simulink model "PID_simulation_kalman"  (R2015b)
settings: Solver=FixedStepAuto  StartTime=0.0  StopTime=10.0  RelTol=1e-3
values from neighbouring files (symbols this model uses):
  P = (eye(2) - K*C)*Pm    [KF.m]    (also in Kalman_filter_7DOF.m; NEW_PID_4DOF.m = PHI*P*PHI' + EE*K*Rb*K'*EE' + Gd; New_PID.m = PHI*P*PHI' + EE*K*Rb*K'*EE' + Gd; P.mat = [1 0 0 0 0 0 0 0 0 0 0 0 ... (3136 elements, 56x56)])
undefined symbols (not defined in the file or in its folder): sample_time
libraries: dspadpt3 x7
settings Model: Creator=Paul_local  LastModifiedBy=Paul_local

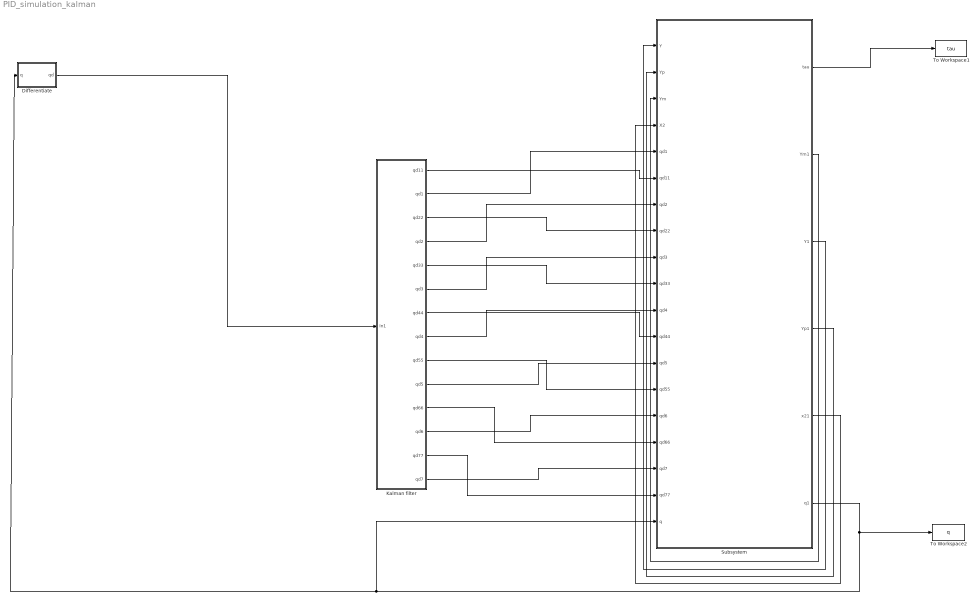
== system PID_simulation_kalman ==
  Differentiate : Subsystem
  Kalman filter : Subsystem
  Subsystem : Subsystem
  To Workspace1 : ToWorkspace  VariableName=tau  SaveFormat=Structure With Time  SampleTime=-1
  To Workspace2 : ToWorkspace  VariableName=q  SaveFormat=Structure With Time  SampleTime=-1
  wires:
  Subsystem/2(Ym1) -> Subsystem/3(Ym)
  Subsystem/5(x21) -> Subsystem/4(X2)
  Subsystem/3(Y1) -> Subsystem/1(Y)
  Subsystem/4(Yp1) -> Subsystem/2(Yp)
  Subsystem/1(tau) -> To Workspace1/1
  Differentiate/1(qd) -> Kalman filter/1(In1)
  Subsystem/6("q1 ") -> To Workspace2/1, Subsystem/19(q), Differentiate/1(q)
  Kalman filter/1(qd11) -> Subsystem/6(qd11)
  Kalman filter/2(qd1) -> Subsystem/5(qd1)
  Kalman filter/3(qd22) -> Subsystem/8(qd22)
  Kalman filter/4(qd2) -> Subsystem/7(qd2)
  Kalman filter/5(qd33) -> Subsystem/10(qd33)
  Kalman filter/6(qd3) -> Subsystem/9(qd3)
  Kalman filter/7(qd44) -> Subsystem/12(qd44)
  Kalman filter/8(qd4) -> Subsystem/11(qd4)
  Kalman filter/9(qd55) -> Subsystem/14(qd55)
  Kalman filter/10(qd5) -> Subsystem/13(qd5)
  Kalman filter/11(qd66) -> Subsystem/16(qd66)
  Kalman filter/12(qd6) -> Subsystem/15(qd6)
  Kalman filter/13(qd77) -> Subsystem/18(qd77)
  Kalman filter/14(qd7) -> Subsystem/17(qd7)

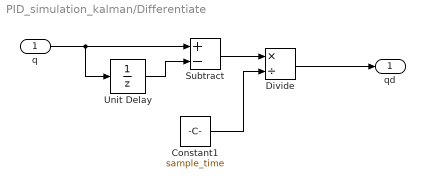
== system PID_simulation_kalman/Differentiate ==
  q : Inport
  Constant1 : Constant  Value=sample_time
  Divide : Product  Inputs=*/
  Subtract : Sum  Inputs=+-
  Unit Delay : UnitDelay  SampleTime=-1
  qd : Outport
  wires:
  q/1 -> Subtract/1, Unit Delay/1
  Unit Delay/1 -> Subtract/2
  Subtract/1 -> Divide/1
  Divide/1 -> qd/1
  Constant1/1 -> Divide/2

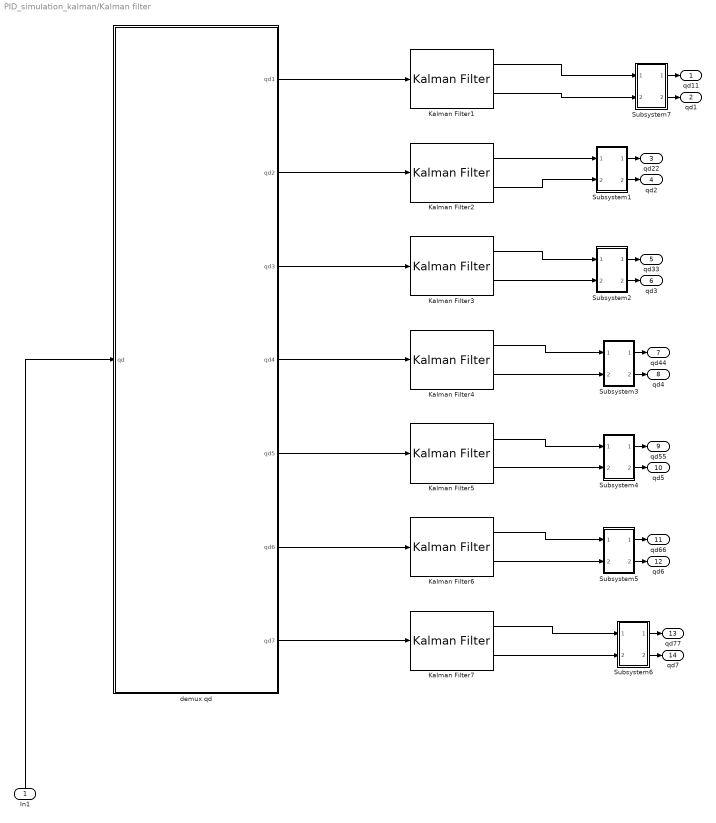
== system PID_simulation_kalman/Kalman filter ==
  In1 : Inport
  Kalman Filter1 : dspadpt3/Kalman Filter  num_targets=1  sourceEnable=Always  isReset=off  X=[-0.1106; 0]  P=[1e-4 0 ; 0 1]  A=[1 0.002 ; 0 1]  sourceMeasure=Specify via Dialog  H=[1 0]  Q=[0 0.000 ;0.000 0.004]  R=1e-5  isOutputEstMeasure=off  isOutputEstState=off  isOutputEstError=off  isOutputPrdMeasure=on  isOutputPrdState=on  isOutputPrdError=off
  Kalman Filter2 : dspadpt3/Kalman Filter  num_targets=1  sourceEnable=Always  isReset=on  X=[-1.94900000000000; 0]  P=[1e-4 0 ; 0 1]  A=[1 0.002 ; 0 1]  sourceMeasure=Specify via Dialog  H=[1 0]  Q=[0 0; 0 0.004]  R=5e-4  isOutputEstMeasure=off  isOutputEstState=off  isOutputEstError=off  isOutputPrdMeasure=on  isOutputPrdState=on  isOutputPrdError=off
  Kalman Filter3 : dspadpt3/Kalman Filter  num_targets=1  sourceEnable=Always  isReset=on  X=[-0.192000000000000; 0]  P=[1e-4 0 ; 0 1]  A=[1 0.002 ; 0 1]  sourceMeasure=Specify via Dialog  H=[1 0]  Q=[0 0; 0 0.004]  R=1e-5  isOutputEstMeasure=off  isOutputEstState=off  isOutputEstError=off  isOutputPrdMeasure=on  isOutputPrdState=on  isOutputPrdError=off
  Kalman Filter4 : dspadpt3/Kalman Filter  num_targets=1  sourceEnable=Always  isReset=on  X=[3.18400000000000; 0]  P=[1e-4 0 ; 0 1]  A=[1 0.002 ; 0 1]  sourceMeasure=Specify via Dialog  H=[1 0]  Q=[0 0; 0 0.004]  R=1e-5  isOutputEstMeasure=off  isOutputEstState=off  isOutputEstError=off  isOutputPrdMeasure=on  isOutputPrdState=on  isOutputPrdError=off
  Kalman Filter5 : dspadpt3/Kalman Filter  num_targets=1  sourceEnable=Always  isReset=on  X=[0.282500000000000; 0]  P=[1e-4 0 ; 0 1]  A=[1 0.002 ; 0 1]  sourceMeasure=Specify via Dialog  H=[1 0]  Q=[0 0; 0 0.004]  R=1e-8  isOutputEstMeasure=off  isOutputEstState=off  isOutputEstError=off  isOutputPrdMeasure=on  isOutputPrdState=on  isOutputPrdError=off
  Kalman Filter6 : dspadpt3/Kalman Filter  num_targets=1  sourceEnable=Always  isReset=on  X=[0.0969000000000000; 0]  P=[1e-4 0 ; 0 1]  A=[1 0.002 ; 0 1]  sourceMeasure=Specify via Dialog  H=[1 0]  Q=[0 0; 0 0.004]  R=1e-8  isOutputEstMeasure=off  isOutputEstState=off  isOutputEstError=off  isOutputPrdMeasure=on  isOutputPrdState=on  isOutputPrdError=off
  Kalman Filter7 : dspadpt3/Kalman Filter  num_targets=1  sourceEnable=Always  isReset=on  X=[-0.279800000000000; 0]  P=[1e-4 0 ; 0 1]  A=[1 0.002 ; 0 1]  sourceMeasure=Specify via Dialog  H=[1 0]  Q=[0 0; 0 0.004]  R=1e-8  isOutputEstMeasure=off  isOutputEstState=off  isOutputEstError=off  isOutputPrdMeasure=on  isOutputPrdState=on  isOutputPrdError=off
  Subsystem1 : Subsystem
  Subsystem2 : Subsystem
  Subsystem3 : Subsystem
  Subsystem4 : Subsystem
  Subsystem5 : Subsystem
  Subsystem6 : Subsystem
  Subsystem7 : Subsystem
  demux qd : Subsystem
  qd11 : Outport
  qd1 : Outport  Port=2
  qd22 : Outport  Port=3
  qd2 : Outport  Port=4
  qd33 : Outport  Port=5
  qd3 : Outport  Port=6
  qd44 : Outport  Port=7
  qd4 : Outport  Port=8
  qd55 : Outport  Port=9
  qd5 : Outport  Port=10
  qd66 : Outport  Port=11
  qd6 : Outport  Port=12
  qd77 : Outport  Port=13
  qd7 : Outport  Port=14
  wires:
  Kalman Filter4/2 -> Subsystem3/2(In2)
  Kalman Filter6/2 -> Subsystem5/2(In2)
  Kalman Filter6/1 -> Subsystem5/1(In1)
  Kalman Filter3/1 -> Subsystem2/1(In1)
  Kalman Filter3/2 -> Subsystem2/2(In2)
  Kalman Filter2/1 -> Subsystem1/1(In1)
  Kalman Filter2/2 -> Subsystem1/2(In2)
  Kalman Filter7/1 -> Subsystem6/1(In1)
  Kalman Filter4/1 -> Subsystem3/1(In1)
  Kalman Filter5/1 -> Subsystem4/1(In1)
  Kalman Filter7/2 -> Subsystem6/2(In2)
  Kalman Filter1/1 -> Subsystem7/1(In1)
  demux qd/5(qd5) -> Kalman Filter5/1
  Kalman Filter5/2 -> Subsystem4/2(In2)
  demux qd/4(qd4) -> Kalman Filter4/1
  demux qd/2(qd2) -> Kalman Filter2/1
  In1/1 -> demux qd/1(qd)
  demux qd/7(qd7) -> Kalman Filter7/1
  demux qd/1(qd1) -> Kalman Filter1/1
  demux qd/3(qd3) -> Kalman Filter3/1
  demux qd/6(qd6) -> Kalman Filter6/1
  Kalman Filter1/2 -> Subsystem7/2(In2)
  Subsystem1/1(qd22) -> qd22/1
  Subsystem7/2(qd1) -> qd1/1
  Subsystem7/1(qd11) -> qd11/1
  Subsystem6/2(qd7) -> qd7/1
  Subsystem4/2(qd5) -> qd5/1
  Subsystem5/2(qd6) -> qd6/1
  Subsystem1/2(qd2) -> qd2/1
  Subsystem2/2(qd3) -> qd3/1
  Subsystem2/1(qd33) -> qd33/1
  Subsystem5/1(qd66) -> qd66/1
  Subsystem6/1(qd77) -> qd77/1
  Subsystem3/1(qd44) -> qd44/1
  Subsystem3/2(qd4) -> qd4/1
  Subsystem4/1(qd55) -> qd55/1

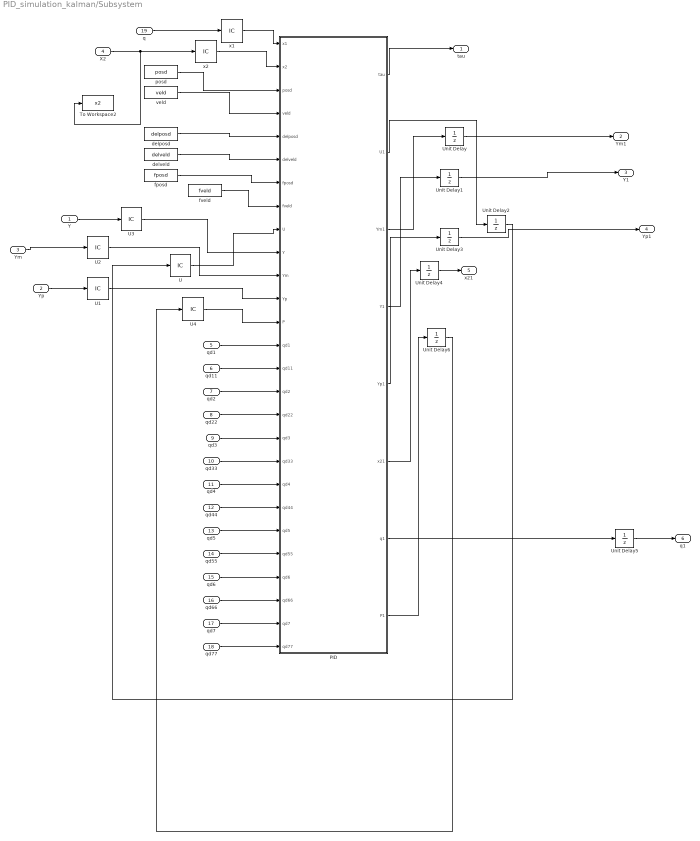
== system PID_simulation_kalman/Subsystem ==
  Y : Inport  PortDimensions=[14]
  Yp : Inport  Port=2  PortDimensions=[14]
  Ym : Inport  Port=3  PortDimensions=[14]
  X2 : Inport  Port=4  PortDimensions=[7]
  qd1 : Inport  Port=5
  qd11 : Inport  Port=6
  qd2 : Inport  Port=7
  qd22 : Inport  Port=8
  qd3 : Inport  Port=9
  qd33 : Inport  Port=10
  qd4 : Inport  Port=11
  qd44 : Inport  Port=12
  qd5 : Inport  Port=13
  qd55 : Inport  Port=14
  qd6 : Inport  Port=15
  qd66 : Inport  Port=16
  qd7 : Inport  Port=17
  qd77 : Inport  Port=18
  q : Inport  Port=19  PortDimensions=[7]
  PID : MATLAB Function  TreatAsAtomicUnit=on
  To Workspace2 : ToWorkspace  VariableName=x2  SaveFormat=Structure With Time  SampleTime=-1
  U : InitialCondition  Value=[0 0 0 0 0 0 0]
  U1 : InitialCondition  Value=[-0.1106,-1.9420,-0.192,3.10200,0.3679,0.1253,-0.3520 0 0 0 0 0 0 0]
  U2 : InitialCondition  Value=[-0.1106,-1.9420,-0.192,3.10200,0.3679,0.1253,-0.3520 0 0 0 0 0 0 0]
  U3 : InitialCondition  Value=[-0.1106,-1.9420,-0.192,3.10200,0.3679,0.1253,-0.3520 0 0 0 0 0 0 0]
  U4 : InitialCondition  Value=P
  Unit Delay : UnitDelay  InitialCondition=[-0.1106,-1.9420,-0.01962,3.10200,0.3679,0.1253,-0.3520 0 0 0 0 0 0 0]  SampleTime=sample_time
  Unit Delay1 : UnitDelay  InitialCondition=[-0.1106,-1.9420,-0.01962,3.10200,0.3679,0.1253,-0.3520 0 0 0 0 0 0 0]  SampleTime=sample_time
  Unit Delay2 : UnitDelay  InitialCondition=[0 0 0 0 0 0 0]  SampleTime=sample_time
  Unit Delay3 : UnitDelay  InitialCondition=[-0.1106,-1.9420,-0.01962,3.10200,0.3679,0.1253,-0.3520 0 0 0 0 0 0 0]  SampleTime=sample_time
  Unit Delay4 : UnitDelay  InitialCondition=zeros(7,1)  SampleTime=sample_time
  Unit Delay5 : UnitDelay  InitialCondition=[-0.1106,-1.9490,-0.0192,3.18400,0.2825,0.0969,-0.2798]  SampleTime=sample_time
  Unit Delay6 : UnitDelay  SampleTime=-1
  "delposd " : FromWorkspace  VariableName=delposd  SampleTime=sample_time
  delveld : FromWorkspace  VariableName=delveld  SampleTime=sample_time
  "fposd " : FromWorkspace  VariableName=fposd  SampleTime=sample_time
  fveld : FromWorkspace  VariableName=fveld  SampleTime=sample_time
  "posd " : FromWorkspace  VariableName=posd  SampleTime=sample_time
  veld : FromWorkspace  VariableName=veld  SampleTime=sample_time
  x1 : InitialCondition  Value=[-0.1106,-1.9490,-0.192,3.18400,0.2825,0.0969,-0.2798]
  x2 : InitialCondition  Value=[0 0 0 0 0 0 0]
  tau : Outport
  Ym1 : Outport  Port=2  PortDimensions=[14]
  Y1 : Outport  Port=3  PortDimensions=[14]
  Yp1 : Outport  Port=4  PortDimensions=[14]
  x21 : Outport  Port=5  PortDimensions=[7]
  "q1 " : Outport  Port=6  PortDimensions=7
  wires:
  x1/1 -> PID/1(x1)
  PID/6(x21) -> Unit Delay4/1
  "delposd "/1 -> PID/5(delposd)
  veld/1 -> PID/4(veld)
  delveld/1 -> PID/6(delveld)
  Y/1 -> U3/1
  x2/1 -> PID/2(x2)
  U3/1 -> PID/10(Y)
  Ym/1 -> U2/1
  Yp/1 -> U1/1
  "posd "/1 -> PID/3(posd)
  Unit Delay2/1 -> U/1
  PID/2(U1) -> Unit Delay2/1
  U/1 -> PID/9(U)
  U2/1 -> PID/11(Ym)
  PID/3(Ym1) -> Unit Delay/1
  fveld/1 -> PID/8(fveld)
  "fposd "/1 -> PID/7(fposd)
  Unit Delay/1 -> Ym1/1
  PID/7(q1) -> Unit Delay5/1
  PID/1(tau) -> tau/1
  U1/1 -> PID/12(Yp)
  X2/1 -> To Workspace2/1, x2/1
  PID/4(Y1) -> Unit Delay1/1
  Unit Delay1/1 -> Y1/1
  Unit Delay3/1 -> Yp1/1
  PID/5(Yp1) -> Unit Delay3/1
  Unit Delay4/1 -> x21/1
  U4/1 -> PID/13(P)
  PID/8(P1) -> Unit Delay6/1
  Unit Delay6/1 -> U4/1
  qd1/1 -> PID/14(qd1)
  qd11/1 -> PID/15(qd11)
  qd2/1 -> PID/16(qd2)
  qd22/1 -> PID/17(qd22)
  qd3/1 -> PID/18(qd3)
  qd33/1 -> PID/19(qd33)
  qd4/1 -> PID/20(qd4)
  qd44/1 -> PID/21(qd44)
  qd5/1 -> PID/22(qd5)
  qd55/1 -> PID/23(qd55)
  qd6/1 -> PID/24(qd6)
  qd66/1 -> PID/25(qd66)
  qd7/1 -> PID/26(qd7)
  qd77/1 -> PID/27(qd77)
  q/1 -> x1/1
  Unit Delay5/1 -> "q1 "/1

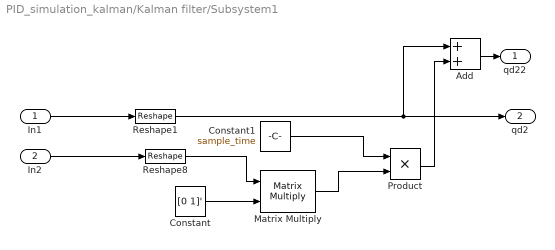
== system PID_simulation_kalman/Kalman filter/Subsystem1 ==
  In1 : Inport
  In2 : Inport  Port=2
  Add : Sum
  Constant : Constant  Value=[0 1]'
  Constant1 : Constant  Value=sample_time
  Matrix Multiply : Product  Multiplication=Matrix(*)
  Product : Product
  Reshape1 : Reshape
  Reshape8 : Reshape  OutputDimensionality=Customize  OutputDimensions=[1,2]
  qd22 : Outport
  qd2 : Outport  Port=2
  wires:
  In2/1 -> Reshape8/1
  Add/1 -> qd22/1
  Product/1 -> Add/2
  In1/1 -> Reshape1/1
  Reshape1/1 -> qd2/1, Add/1
  Matrix Multiply/1 -> Product/2
  Constant/1 -> Matrix Multiply/2
  Constant1/1 -> Product/1
  Reshape8/1 -> Matrix Multiply/1

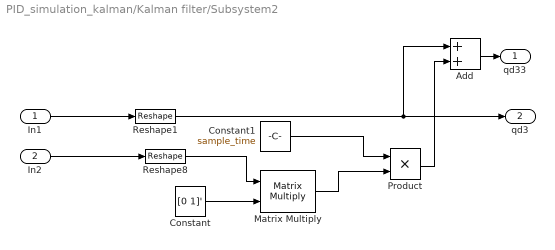
== system PID_simulation_kalman/Kalman filter/Subsystem2 ==
  In1 : Inport
  In2 : Inport  Port=2
  Add : Sum
  Constant : Constant  Value=[0 1]'
  Constant1 : Constant  Value=sample_time
  Matrix Multiply : Product  Multiplication=Matrix(*)
  Product : Product
  Reshape1 : Reshape
  Reshape8 : Reshape  OutputDimensionality=Customize  OutputDimensions=[1,2]
  qd33 : Outport
  qd3 : Outport  Port=2
  wires:
  In2/1 -> Reshape8/1
  Add/1 -> qd33/1
  Product/1 -> Add/2
  In1/1 -> Reshape1/1
  Reshape1/1 -> qd3/1, Add/1
  Matrix Multiply/1 -> Product/2
  Constant/1 -> Matrix Multiply/2
  Constant1/1 -> Product/1
  Reshape8/1 -> Matrix Multiply/1

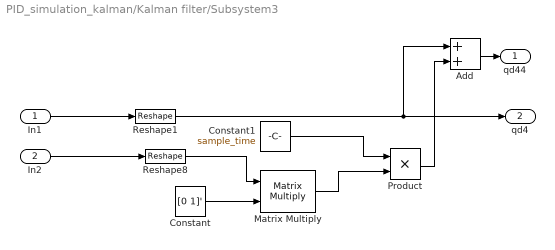
== system PID_simulation_kalman/Kalman filter/Subsystem3 ==
  In1 : Inport
  In2 : Inport  Port=2
  Add : Sum
  Constant : Constant  Value=[0 1]'
  Constant1 : Constant  Value=sample_time
  Matrix Multiply : Product  Multiplication=Matrix(*)
  Product : Product
  Reshape1 : Reshape
  Reshape8 : Reshape  OutputDimensionality=Customize  OutputDimensions=[1,2]
  qd44 : Outport
  qd4 : Outport  Port=2
  wires:
  In2/1 -> Reshape8/1
  Add/1 -> qd44/1
  Product/1 -> Add/2
  In1/1 -> Reshape1/1
  Reshape1/1 -> qd4/1, Add/1
  Matrix Multiply/1 -> Product/2
  Constant/1 -> Matrix Multiply/2
  Constant1/1 -> Product/1
  Reshape8/1 -> Matrix Multiply/1

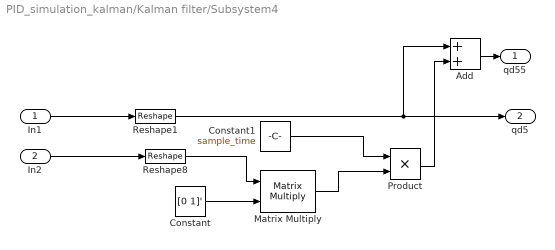
== system PID_simulation_kalman/Kalman filter/Subsystem4 ==
  In1 : Inport
  In2 : Inport  Port=2
  Add : Sum
  Constant : Constant  Value=[0 1]'
  Constant1 : Constant  Value=sample_time
  Matrix Multiply : Product  Multiplication=Matrix(*)
  Product : Product
  Reshape1 : Reshape
  Reshape8 : Reshape  OutputDimensionality=Customize  OutputDimensions=[1,2]
  qd55 : Outport
  qd5 : Outport  Port=2
  wires:
  In2/1 -> Reshape8/1
  Add/1 -> qd55/1
  Product/1 -> Add/2
  In1/1 -> Reshape1/1
  Reshape1/1 -> qd5/1, Add/1
  Matrix Multiply/1 -> Product/2
  Constant/1 -> Matrix Multiply/2
  Constant1/1 -> Product/1
  Reshape8/1 -> Matrix Multiply/1

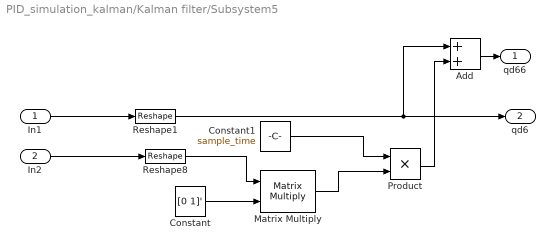
== system PID_simulation_kalman/Kalman filter/Subsystem5 ==
  In1 : Inport
  In2 : Inport  Port=2
  Add : Sum
  Constant : Constant  Value=[0 1]'
  Constant1 : Constant  Value=sample_time
  Matrix Multiply : Product  Multiplication=Matrix(*)
  Product : Product
  Reshape1 : Reshape
  Reshape8 : Reshape  OutputDimensionality=Customize  OutputDimensions=[1,2]
  qd66 : Outport
  qd6 : Outport  Port=2
  wires:
  In2/1 -> Reshape8/1
  Add/1 -> qd66/1
  Product/1 -> Add/2
  In1/1 -> Reshape1/1
  Reshape1/1 -> qd6/1, Add/1
  Matrix Multiply/1 -> Product/2
  Constant/1 -> Matrix Multiply/2
  Constant1/1 -> Product/1
  Reshape8/1 -> Matrix Multiply/1

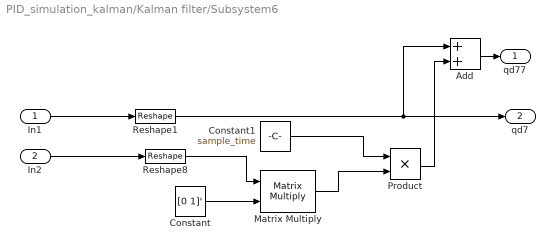
== system PID_simulation_kalman/Kalman filter/Subsystem6 ==
  In1 : Inport
  In2 : Inport  Port=2
  Add : Sum
  Constant : Constant  Value=[0 1]'
  Constant1 : Constant  Value=sample_time
  Matrix Multiply : Product  Multiplication=Matrix(*)
  Product : Product
  Reshape1 : Reshape
  Reshape8 : Reshape  OutputDimensionality=Customize  OutputDimensions=[1,2]
  qd77 : Outport
  qd7 : Outport  Port=2
  wires:
  In2/1 -> Reshape8/1
  Add/1 -> qd77/1
  Product/1 -> Add/2
  In1/1 -> Reshape1/1
  Reshape1/1 -> qd7/1, Add/1
  Matrix Multiply/1 -> Product/2
  Constant/1 -> Matrix Multiply/2
  Constant1/1 -> Product/1
  Reshape8/1 -> Matrix Multiply/1

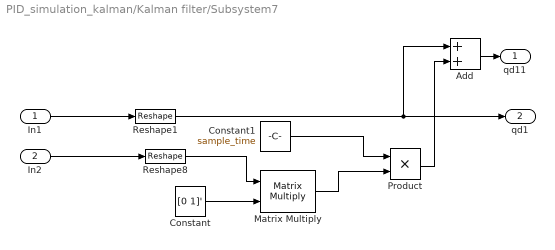
== system PID_simulation_kalman/Kalman filter/Subsystem7 ==
  In1 : Inport
  In2 : Inport  Port=2
  Add : Sum
  Constant : Constant  Value=[0 1]'
  Constant1 : Constant  Value=sample_time
  Matrix Multiply : Product  Multiplication=Matrix(*)
  Product : Product
  Reshape1 : Reshape
  Reshape8 : Reshape  OutputDimensionality=Customize  OutputDimensions=[1,2]
  qd11 : Outport
  qd1 : Outport  Port=2
  wires:
  In2/1 -> Reshape8/1
  Add/1 -> qd11/1
  Product/1 -> Add/2
  In1/1 -> Reshape1/1
  Reshape1/1 -> qd1/1, Add/1
  Matrix Multiply/1 -> Product/2
  Constant/1 -> Matrix Multiply/2
  Constant1/1 -> Product/1
  Reshape8/1 -> Matrix Multiply/1

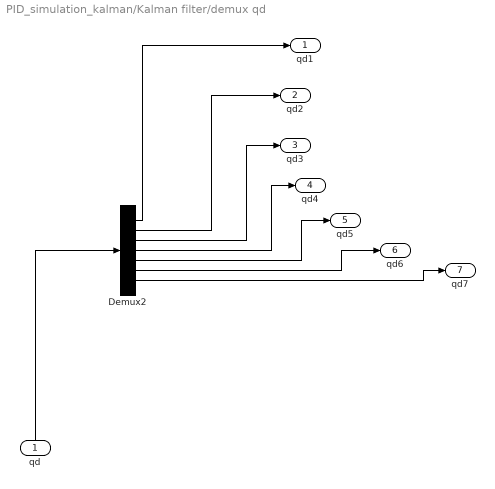
== system PID_simulation_kalman/Kalman filter/demux qd ==
  qd : Inport
  Demux2 : Demux  Outputs=7
  qd1 : Outport
  qd2 : Outport  Port=2
  qd3 : Outport  Port=3
  qd4 : Outport  Port=4
  qd5 : Outport  Port=5
  qd6 : Outport  Port=6
  qd7 : Outport  Port=7
  wires:
  qd/1 -> Demux2/1
  Demux2/1 -> qd1/1
  Demux2/2 -> qd2/1
  Demux2/3 -> qd3/1
  Demux2/4 -> qd4/1
  Demux2/5 -> qd5/1
  Demux2/6 -> qd6/1
  Demux2/7 -> qd7/1

== matlab function PID_simulation_kalman/Subsystem/PID ==
  data: x1 input; x2 input; posd input; tau output; veld input; delposd input; delveld input; fposd input; fveld input; U input; U1 output; Ym1 output; Y1 output; Yp1 output; x21 output; Y input; Ym input; Yp input; q1 output; P input; P1 output; qd1 input; qd11 input; qd2 input; qd22 input; qd3 input; qd33 input; qd4 input; qd44 input; qd5 input; qd55 input; qd6 input; qd66 input; qd7 input; qd77 input
%
% gravComp7DOFNum Compute inverse dynamics via recursive Newton-Euler formulation
%
% Recursive Newton-Euler for standard Denavit-Hartenberg notation.
%

% Copyright (C) 1993-2011, by Peter I. Corke
%
% This file originally was part of The Robotics Toolbox for Matlab (RTB).
%
% http://www.petercorke.com

%
% Simplified from rne_dh for 7DOF WAM to compute only torque from gravity by Hans Vorsteveld
% Does not use structures from RTB, only the RNE algorithm
%

function [tau,U1,Ym1,Y1,Yp1,x21,q1,P1] = PID(x1,x2,posd,veld,delposd,delveld,fposd,fveld,U,Y,Ym,Yp,P,qd1,qd11,qd2,qd22,qd3,qd33,qd4,qd44,qd5,qd55,qd6,qd66,qd7,qd77)

%-------------------------------------------------------------------------------------
%   SETUP THE ARM
%-------------------------------------------------------------------------------------    
    n = 14;p = 7; q = 14;
    
 Ts=0.01; 


 
 


yddel=[delposd;delveld];
yd = [posd;veld];
fyd=[fposd;fveld];


 

%initial conditions
%x1 = [-0.11060;-1.949;-0.1920;3.1840;0.2825;0.09690;-0.27980];
%x2 = zeros(7,1);
%U = zeros(7,1);
Ae = 0.9*eye(n);
C= eye(14);
Ce = C;
Iq = eye(q);
Oq = zeros(q);
H = [Iq Oq Oq -Ce*Ae;Iq Oq Oq zeros(q,n);Oq Iq Oq zeros(q,n);zeros(n,q) zeros(n,q) zeros(n,q) Ae];
Ib = zeros(3*q,3*q+n);
for k11 = 1:3*q,Ib(k11,k11) = 1;end
sig = 1e-3;
sigR = sig;
sigQ = 1e-4;%1e-3;
alfa = 1e0;
beta = 1e-2;
p1 = alfa*ones(1,3*q);
p2 = beta*ones(1,n);
pb = [p1 p2];

r1 = 5;
r2 = 50;
r3 = 1.5;
rv = 10;
rbb1 = r1*sig^2*ones(1,q/2);
rbb2 = r2*0.1*sig^2*ones(1,q/2);
rbb12 = [rbb1 rbb2];
rbb = [r3*rbb12 rbb12 rbb12];
 
Rb = 1*diag(rbb);
Q = 0*sigQ^2*eye(n);





 Be = Ts*[zeros(7,7);inv(D(x1))];
    Delyd=[fyd-yd];
    Del2yd = Delyd*Delyd';
   
    Gd = [Del2yd Oq Oq zeros(q,n); Oq Oq Oq zeros(q,n); Oq Oq Oq zeros(q,n);zeros(n,q) zeros(n,q) zeros(n,q) Q];
   
    
    
    EE = [Ce*Be;zeros(q,p);zeros(q,p);-Be];
    K = inv(EE'*EE)*EE'*H*P*Ib'*inv(Ib*P*Ib' + Rb);
    PHI = H - EE*K*Ib;

    P1 = PHI*P*PHI' + EE*K*Rb*K'*EE' + Gd;
    K1 = K(:,1:q);
    K2 = K(:,q+1:2*q);
    K3 = K(:,2*q+1:3*q);
    
    
      %  E = yd - Y ;
       % Ep = ydfut-Yp ;
        %U = U + K1*Ep + K2*E;
        %Ym = Y;
        %Y = Yp;
         %x_1 = x1 ;
       
         %x_11 = x_1; %Since at t=0, velocity is zero
        %XX2 = zeros(7,1);
        %x_22= (-inv(D(x_1))*(transpose(G(x_1)))+ inv(D(x_1))*U)*Ts + XX2 ;
        %Yp = [x_11' x_22']';
       
    
        Em = yddel - Ym ;
        E = yd - Y ;
        Ep = fyd-Yp ;
        U = U + K1*Ep + K2*E + K3*Em;
        Ym = Y;
        Y = Yp;
        
        
        x2=[qd1;qd2;qd3;qd4;qd5;qd6;qd7];
        
         %
        pos_meas = x1 ; % In experimental work you do not add noise instead you only use measurement of position
        x_11 =  x2*Ts + pos_meas; % Here we are estimating position using the extimate of x2 and measurement of x1 at present time
        
        %XX2 = (x_11-x_1)/Ts; 
        %XX2 = (x1-x1d)/Ts; 
        
        %x_22= (-inv(D(pos_meas))*((G(pos_meas)))+ inv(D(pos_meas))*U)*Ts + XX2 ;
        x_22=[qd11;qd22;qd33;qd44;qd55;qd66;qd77];
        
        Yp = [x_11' x_22']';
        q1=x_11;
        tau=U;
        Yp1=Yp;
        Ym1=Ym;
        Y1=Y;
        U1=U;
        x21= x_22;
    
   
end 

function G = G(q)

DH_a = [0 0 0.045 -0.045 0 0 0];
    DH_d = [0 0 .55 0 0.3 0 0.061];
    DH_alpha = [-pi/2 pi/2 -pi/2 pi/2 -pi/2 pi/2 0];
 
    m = [10.7676 3.87 1.8022 2.4 0.1237 0.4979886 0.07548270];
    
    com = zeros(3,7);
    com(:,1) = [-0.00443422; 0.12189039; -0.00066489];
    com(:,2) = [-0.00236983; 0.03105614; 0.01542114 ];
    com(:,3) = [-0.03825858; 0.20750770; 0.00003309];
    com(:,4) = [ 0.00498512;-0.00022942;0.13271662 ];
    com(:,5) = [0.00008921;0.00511217;0.00435824];
    com(:,6) = [-0.00012262;-0.01703194;0.02468336];
    com(:,7) = [-0.00007974;0.00016313;-0.00323552 ];
     
    
    T = zeros(4,4,7);
     
for j=1:7,
        a = DH_a(j);
        d = DH_d(j);
        alpha = DH_alpha(j);
        T(:,:,j) = getTransformDH(a, d, alpha, q(j));
end 
comstar = zeros(4,7);
    comstar(:,1) = [com(:,1);1];
    comstar(:,2) = [com(:,2);1];
    comstar(:,3) = [com(:,3);1];
    comstar(:,4) = [com(:,4);1];
    comstar(:,5) = [com(:,5);1];
    comstar(:,6) = [com(:,6);1];
    comstar(:,7) = [ com(:,7);1];
  
    Q=[0,-1,0,0;
     1,0,0,0;
     0,0,0,0;
     0,0,0,0];
   
 gravity=[0,0,-9.81,0];
 G=zeros(7,1);
 
   G(1)= -m(1)*gravity*Q*T(:,:,1)*comstar(:,1)-m(2)*gravity*Q*T(:,:,1)*T(:,:,2)*comstar(:,2)-m(3)*gravity*Q*T(:,:,1)*T(:,:,2)*T(:,:,3)*comstar(:,3)-m(4)*gravity*Q*T(:,:,1)*T(:,:,2)*T(:,:,3)*T(:,:,4)*comstar(:,4)-m(5)*gravity*Q*T(:,:,1)*T(:,:,2)*T(:,:,3)*T(:,:,4)*T(:,:,5)*comstar(:,5)-m(6)*gravity*Q*T(:,:,1)*T(:,:,2)*T(:,:,3)*T(:,:,4)*T(:,:,5)*T(:,:,6)*comstar(:,6)-m(7)*gravity*Q*T(:,:,1)*T(:,:,2)*T(:,:,3)*T(:,:,4)*T(:,:,5)*T(:,:,6)*T(:,:,7)*comstar(:,7);   
   G(2)= -m(2)*gravity*T(:,:,1)*Q*T(:,:,2)*comstar(:,2)-m(3)*gravity*T(:,:,1)*Q*T(:,:,2)*T(:,:,3)*comstar(:,3)-m(4)*gravity*T(:,:,1)*Q*T(:,:,2)*T(:,:,3)*T(:,:,4)*comstar(:,4)-m(5)*gravity*T(:,:,1)*Q*T(:,:,2)*T(:,:,3)*T(:,:,4)*T(:,:,5)*comstar(:,5)-m(6)*gravity*T(:,:,1)*Q*T(:,:,2)*T(:,:,3)*T(:,:,4)*T(:,:,5)*T(:,:,6)*comstar(:,6)-m(7)*gravity*T(:,:,1)*Q*T(:,:,2)*T(:,:,3)*T(:,:,4)*T(:,:,5)*T(:,:,6)*T(:,:,7)*comstar(:,7);
   G(3)= -m(3)*gravity*T(:,:,1)*T(:,:,2)*Q*T(:,:,3)*comstar(:,3)-m(4)*gravity*T(:,:,1)*T(:,:,2)*Q*T(:,:,3)*T(:,:,4)*comstar(:,4)-m(5)*gravity*T(:,:,1)*T(:,:,2)*Q*T(:,:,3)*T(:,:,4)*T(:,:,5)*comstar(:,5)-m(6)*gravity*T(:,:,1)*T(:,:,2)*Q*T(:,:,3)*T(:,:,4)*T(:,:,5)*T(:,:,6)*comstar(:,6)-m(7)*gravity*T(:,:,1)*T(:,:,2)*Q*T(:,:,3)*T(:,:,4)*T(:,:,5)*T(:,:,6)*T(:,:,7)*comstar(:,7);
   G(4)= -m(4)*gravity*T(:,:,1)*T(:,:,2)*T(:,:,3)*Q*T(:,:,4)*comstar(:,4)-m(5)*gravity*T(:,:,1)*T(:,:,2)*T(:,:,3)*Q*T(:,:,4)*T(:,:,5)*comstar(:,5)-m(6)*gravity*T(:,:,1)*T(:,:,2)*T(:,:,3)*Q*T(:,:,4)*T(:,:,5)*T(:,:,6)*comstar(:,6)-m(7)*gravity*T(:,:,1)*T(:,:,2)*T(:,:,3)*Q*T(:,:,4)*T(:,:,5)*T(:,:,6)*T(:,:,7)*comstar(:,7);
   G(5)= -m(5)*gravity*T(:,:,1)*T(:,:,2)*T(:,:,3)*T(:,:,4)*Q*T(:,:,5)*comstar(:,5)-m(6)*gravity*T(:,:,1)*T(:,:,2)*T(:,:,3)*T(:,:,4)*Q*T(:,:,5)*T(:,:,6)*comstar(:,6)-m(7)*gravity*T(:,:,1)*T(:,:,2)*T(:,:,3)*T(:,:,4)*Q*T(:,:,5)*T(:,:,6)*T(:,:,7)*comstar(:,7);
   G(6)= -m(6)*gravity*T(:,:,1)*T(:,:,2)*T(:,:,3)*T(:,:,4)*T(:,:,5)*Q*T(:,:,6)*comstar(:,6)-m(7)*gravity*T(:,:,1)*T(:,:,2)*T(:,:,3)*T(:,:,4)*T(:,:,5)*Q*T(:,:,6)*T(:,:,7)*comstar(:,7);
   G(7)= -m(7)*gravity*T(:,:,1)*T(:,:,2)*T(:,:,3)*T(:,:,4)*T(:,:,5)*T(:,:,6)*Q*T(:,:,7)*comstar(:,7);
   
end 
function bq = bq(qd)
 
 
 
s=20;
bc = [2.516; 2.581; 2.038; 0.956; 0.323; 0.315; 0.066];
B =  [1.142; 0.946; 0.309; 0.255; 0.025; 0.039; 0.004];
 
bq = bc.*atan(s*qd)*2/pi+B.*qd;
end 

function D =D(q)
DH_a = [0 0 0.045 -0.045 0 0 0];
    DH_d = [0 0 .55 0 0.3 0 0.061];
    DH_alpha = [-pi/2 pi/2 -pi/2 pi/2 -pi/2 pi/2 0];
 
    m = [10.7676 3.87 1.8022 2.4 0.1237 0.4179886 0.07548270];
    
     
    
    com = zeros(3,7);
   com(:,1) = [-0.00443422; 0.12189039; -0.00066489];
    com(:,2) = [-0.00236983; 0.03105614; 0.01542114 ];
    com(:,3) = [-0.03825858; 0.20750770; 0.00003309];
    com(:,4) = [ 0.00498512;-0.00022942;0.13271662 ];
    com(:,5) = [0.00008921;0.00511217;0.00435824];
    com(:,6) = [-0.00012262;-0.01703194;0.02468336];
    com(:,7) = [-0.00007974;0.00016313;-0.00323552 ];
     
    I=zeros(3,3,7);
    
     I(:,:,1) = [ 0.29486350 , -0.00795023 ,-0.00009311;
                 -0.00795023 , 0.11350017 , -0.00018711;
                -0.00009311 , -0.00018711 , 0.25065343];
    I(:,:,2) =[0.02606840 ,-0.00001346 , -0.00011701;
               -0.00001346,  0.01472202 ,0.00003659;
               -0.00011701 , 0.00003659,  0.01934814];
    I(:,:,3) = [0.13671601,  -0.01680434,  0.00000510;
               -0.01680434 , 0.00588354 , -0.00000530;
                0.00000510 , -0.00000530 , 0.13951371];
    I(:,:,4) = [ 0.05719268 , 0.00001467 , 0.00008193;
                 0.00001467 , 0.05716470 , -0.00009417;
                 0.00008193 , -0.00009417 , 0.00300441] ;
    I(:,:,5) =[0.00005587 , 0.00000026,  0.00000000;
               0.00000026 , 0.00007817,  -0.00000083;
               0.00000000 , -0.00000083,  0.00006594];
    I(:,:,6) = [0.00093106,  0.00000148 , -0.00000201;
                0.00000148,  0.00049833 , -0.00022162;
               -0.00000201,  -0.00022162,  0.00057483];
   I(:,:,7) = [0.00003845,  -0.00000019 , 0.00000002;
                -0.00000019, 0.00003878 , -0.00000004;
                0.00000002 ,  -0.00000004, 0.00007408 ];
            T=zeros(4,4,7);
  
             
for j=1:7,
        a = DH_a(j);
        d = DH_d(j);
        alpha = DH_alpha(j);
        T(:,:,j) = getTransformDH(a, d, alpha, q(j));
end 
 
 
 
 
   comstar = zeros(4,7);
    comstar(:,1) = [com(:,1);1];
    comstar(:,2) = [com(:,2);1];
    comstar(:,3) = [com(:,3);1];
    comstar(:,4) = [com(:,4);1];
    comstar(:,5) = [com(:,5);1];
    comstar(:,6) = [com(:,6);1];
    comstar(:,7) = [ com(:,7);1];
  
    Q=[0,-1,0,0;
     1,0,0,0;
     0,0,0,0;
     0,0,0,0];
   
U=zeros(4,4,7,7);
   U(:,:,1,1)= Q*T(:,:,1);
   U(:,:,2,1)= Q*T(:,:,1)*T(:,:,2);
   U(:,:,3,1)= Q*T(:,:,1)*T(:,:,2)*T(:,:,3);
   U(:,:,4,1)= Q*T(:,:,1)*T(:,:,2)*T(:,:,3)*T(:,:,4);
   U(:,:,5,1)= Q*T(:,:,1)*T(:,:,2)*T(:,:,3)*T(:,:,4)*T(:,:,5);
   U(:,:,6,1)= Q*T(:,:,1)*T(:,:,2)*T(:,:,3)*T(:,:,4)*T(:,:,5)*T(:,:,6);
   U(:,:,7,1)= Q*T(:,:,1)*T(:,:,2)*T(:,:,3)*T(:,:,4)*T(:,:,5)*T(:,:,6)*T(:,:,7);
   
   
   U(:,:,2,2)= T(:,:,1)*Q*T(:,:,2);
   U(:,:,3,2)= T(:,:,1)*Q*T(:,:,2)*T(:,:,3);
   U(:,:,4,2)= T(:,:,1)*Q*T(:,:,2)*T(:,:,3)*T(:,:,4);
   U(:,:,5,2)= T(:,:,1)*Q*T(:,:,2)*T(:,:,3)*T(:,:,4)*T(:,:,5);
   U(:,:,6,2)= T(:,:,1)*Q*T(:,:,2)*T(:,:,3)*T(:,:,4)*T(:,:,5)*T(:,:,6);
   U(:,:,7,2)= T(:,:,1)*Q*T(:,:,2)*T(:,:,3)*T(:,:,4)*T(:,:,5)*T(:,:,6)*T(:,:,7);
   
  
   U(:,:,3,3)= T(:,:,1)*T(:,:,2)*Q*T(:,:,3);
   U(:,:,4,3)= T(:,:,1)*T(:,:,2)*Q*T(:,:,3)*T(:,:,4);
   U(:,:,5,3)= T(:,:,1)*T(:,:,2)*Q*T(:,:,3)*T(:,:,4)*T(:,:,5);
   U(:,:,6,3)= T(:,:,1)*T(:,:,2)*Q*T(:,:,3)*T(:,:,4)*T(:,:,5)*T(:,:,6);
   U(:,:,7,3)= T(:,:,1)*T(:,:,2)*Q*T(:,:,3)*T(:,:,4)*T(:,:,5)*T(:,:,6)*T(:,:,7);
   
   U(:,:,4,4)= T(:,:,1)*T(:,:,2)*T(:,:,3)*Q*T(:,:,4);
   U(:,:,5,4)= T(:,:,1)*T(:,:,2)*T(:,:,3)*Q*T(:,:,4)*T(:,:,5);
   U(:,:,6,4)= T(:,:,1)*T(:,:,2)*T(:,:,3)*Q*T(:,:,4)*T(:,:,5)*T(:,:,6);
   U(:,:,7,4)= T(:,:,1)*T(:,:,2)*T(:,:,3)*Q*T(:,:,4)*T(:,:,5)*T(:,:,6)*T(:,:,7);
   
   U(:,:,5,5)= T(:,:,1)*T(:,:,2)*T(:,:,3)*T(:,:,4)*Q*T(:,:,5);
   U(:,:,6,5)= T(:,:,1)*T(:,:,2)*T(:,:,3)*T(:,:,4)*Q*T(:,:,5)*T(:,:,6);
   U(:,:,7,5)= T(:,:,1)*T(:,:,2)*T(:,:,3)*T(:,:,4)*Q*T(:,:,5)*T(:,:,6)*T(:,:,7);
   
   U(:,:,6,6)= T(:,:,1)*T(:,:,2)*T(:,:,3)*T(:,:,4)*T(:,:,5)*Q*T(:,:,6);
   U(:,:,7,6)= T(:,:,1)*T(:,:,2)*T(:,:,3)*T(:,:,4)*T(:,:,5)*Q*T(:,:,6)*T(:,:,7);
   
   U(:,:,7,7)= T(:,:,1)*T(:,:,2)*T(:,:,3)*T(:,:,4)*T(:,:,5)*T(:,:,6)*Q*T(:,:,7);
   
   
   
  
   J=zeros(4,4,7);
 
   
   J(:,:,1)=[0.5*(-I(1,1,1)+I(2,2,1)+I(3,3,1)), I(1,2,1), I(1,3,1), m(1)*com(1,1);
             I(1,2,1) ,0.5*(I(1,1,1)-I(2,2,1)+I(3,3,1)), I(2,3,1), m(1)*com(2,1);
             I(1,3,1), I(2,3,1), 0.5*(I(1,1,1)+I(2,2,1)-I(3,3,1)), m(1)*com(3,1);
              m(1)*com(1,1), m(1)*com(2,1), m(1)*com(3,1), m(1)];
   
    J(:,:,2)=[0.5*(-I(1,1,2)+I(2,2,2)+I(3,3,2)), I(1,2,2), I(1,3,2), m(2)*com(1,2);
             I(1,2,2) ,0.5*(I(1,1,2)-I(2,2,2)+I(3,3,2)), I(2,3,2), m(2)*com(2,2);
             I(1,3,2), I(2,3,2), 0.5*(I(1,1,2)+I(2,2,2)-I(3,3,2)), m(2)*com(3,2);
              m(2)*com(1,2), m(2)*com(2,2), m(2)*com(3,2), m(2)];
   
          
     J(:,:,3)=[0.5*(-I(1,1,3)+I(2,2,3)+I(3,3,3)), I(1,2,3), I(1,3,3), m(3)*com(1,3);
             I(1,2,3) ,0.5*(I(1,1,3)-I(2,2,3)+I(3,3,3)), I(2,3,3), m(3)*com(2,3);
             I(1,3,3), I(2,3,3), 0.5*(I(1,1,3)+I(2,2,3)-I(3,3,3)), m(3)*com(3,3);
              m(3)*com(1,3), m(3)*com(2,3), m(3)*com(3,3), m(3)];      
   
   
    J(:,:,4)=[0.5*(-I(1,1,4)+I(2,2,4)+I(3,3,4)), I(1,2,4), I(1,3,4), m(4)*com(1,4);
             I(1,2,4) ,0.5*(I(1,1,4)-I(2,2,4)+I(3,3,4)), I(2,3,4), m(4)*com(2,4);
             I(1,3,4), I(2,3,4), 0.5*(I(1,1,4)+I(2,2,4)-I(3,3,4)), m(4)*com(3,4);
              m(4)*com(1,4), m(4)*com(2,4), m(4)*com(3,4), m(4)];
   
   
    J(:,:,5)=[0.5*(-I(1,1,5)+I(2,2,5)+I(3,3,5)), I(1,2,5), I(1,3,5), m(5)*com(1,5);
             I(1,2,5) ,0.5*(I(1,1,5)-I(2,2,5)+I(3,3,5)), I(2,3,5), m(5)*com(2,5);
             I(1,3,5), I(2,3,5), 0.5*(I(1,1,5)+I(2,2,5)-I(3,3,5)), m(5)*com(3,5);
              m(5)*com(1,5), m(5)*com(2,5), m(5)*com(3,5), m(5)];
   
   
    J(:,:,6)=[0.5*(-I(1,1,6)+I(2,2,6)+I(3,3,6)), I(1,2,6), I(1,3,6), m(6)*com(1,6);
             I(1,2,6) ,0.5*(I(1,1,6)-I(2,2,6)+I(3,3,6)), I(2,3,6), m(6)*com(2,6);
             I(1,3,6), I(2,3,6), 0.5*(I(1,1,6)+I(2,2,6)-I(3,3,6)), m(6)*com(3,6);
              m(6)*com(1,6), m(6)*com(2,6), m(6)*com(3,6), m(6)];
   
   
    J(:,:,7)=[0.5*(-I(1,1,7)+I(2,2,7)+I(3,3,7)), I(1,2,7), I(1,3,7), m(7)*com(1,7);
             I(1,2,7) ,0.5*(I(1,1,7)-I(2,2,7)+I(3,3,7)), I(2,3,7), m(7)*com(2,7);
             I(1,3,7), I(2,3,7), 0.5*(I(1,1,7)+I(2,2,7)-I(3,3,7)), m(7)*com(3,7);
              m(7)*com(1,7), m(7)*com(2,7), m(7)*com(3,7), m(7)];
   
   D=zeros(7,7);
    D(1,1)= trace(U(:,:,1,1)*J(:,:,1)*transpose(U(:,:,1,1))) + trace(U(:,:,2,1)*J(:,:,2)*transpose(U(:,:,2,1))) + trace(U(:,:,3,1)*J(:,:,3)*transpose(U(:,:,3,1))) + trace(U(:,:,4,1)*J(:,:,4)*transpose(U(:,:,4,1))) + trace(U(:,:,5,1)*J(:,:,5)*transpose(U(:,:,5,1))) + trace(U(:,:,6,1)*J(:,:,6)*transpose(U(:,:,6,1))) + trace(U(:,:,7,1)*J(:,:,7)*transpose(U(:,:,7,1))) ;
    D(1,2)= trace(U(:,:,2,2)*J(:,:,2)*transpose(U(:,:,2,1))) + trace(U(:,:,3,2)*J(:,:,3)*transpose(U(:,:,3,1))) + trace(U(:,:,4,2)*J(:,:,4)*transpose(U(:,:,4,1))) +trace(U(:,:,5,2)*J(:,:,5)*transpose(U(:,:,5,1))) + trace(U(:,:,6,2)*J(:,:,6)*transpose(U(:,:,6,1))) + trace(U(:,:,7,2)*J(:,:,7)*transpose(U(:,:,7,1))); 
    D(1,3)= trace(U(:,:,3,3)*J(:,:,3)*transpose(U(:,:,3,1)))+ trace(U(:,:,4,3)*J(:,:,4)*transpose(U(:,:,4,1)))+ trace(U(:,:,5,3)*J(:,:,5)*transpose(U(:,:,5,1)))+ trace(U(:,:,6,3)*J(:,:,6)*transpose(U(:,:,6,1)))+ trace(U(:,:,7,3)*J(:,:,7)*transpose(U(:,:,7,1))); 
    D(1,4)= trace(U(:,:,4,4)*J(:,:,4)*transpose(U(:,:,4,1)))+ trace(U(:,:,5,4)*J(:,:,5)*transpose(U(:,:,5,1)))+ trace(U(:,:,6,4)*J(:,:,6)*transpose(U(:,:,6,1)))+ trace(U(:,:,7,4)*J(:,:,7)*transpose(U(:,:,7,1)));
    D(1,5)= trace(U(:,:,5,5)*J(:,:,5)*transpose(U(:,:,5,1)))+ trace(U(:,:,6,5)*J(:,:,6)*transpose(U(:,:,6,1)))+ trace(U(:,:,7,5)*J(:,:,7)*transpose(U(:,:,7,1)));
    D(1,6)= trace(U(:,:,6,6)*J(:,:,6)*transpose(U(:,:,6,1)))+ trace(U(:,:,7,6)*J(:,:,7)*transpose(U(:,:,7,1)));
    D(1,7)= trace(U(:,:,7,7)*J(:,:,7)*transpose(U(:,:,7,1)));
    
    D(2,1)= trace(U(:,:,2,1)*J(:,:,2)*transpose(U(:,:,2,2)))+ trace(U(:,:,3,1)*J(:,:,3)*transpose(U(:,:,3,2)))+ trace(U(:,:,4,1)*J(:,:,4)*transpose(U(:,:,4,2)))+ trace(U(:,:,5,1)*J(:,:,5)*transpose(U(:,:,5,2)))+ trace(U(:,:,6,1)*J(:,:,6)*transpose(U(:,:,6,2)))+ trace(U(:,:,7,1)*J(:,:,7)*transpose(U(:,:,7,2)));
    D(2,2)= trace(U(:,:,2,2)*J(:,:,2)*transpose(U(:,:,2,2)))+ trace(U(:,:,3,2)*J(:,:,3)*transpose(U(:,:,3,2)))+ trace(U(:,:,4,2)*J(:,:,4)*transpose(U(:,:,4,2)))+ trace(U(:,:,5,2)*J(:,:,5)*transpose(U(:,:,5,2)))+ trace(U(:,:,6,2)*J(:,:,6)*transpose(U(:,:,6,2)))+ trace(U(:,:,7,2)*J(:,:,7)*transpose(U(:,:,7,2)));
    D(2,3)= trace(U(:,:,3,3)*J(:,:,3)*transpose(U(:,:,3,2)))+ trace(U(:,:,4,3)*J(:,:,4)*transpose(U(:,:,4,2)))+ trace(U(:,:,5,3)*J(:,:,5)*transpose(U(:,:,5,2)))+ trace(U(:,:,6,3)*J(:,:,6)*transpose(U(:,:,6,2)))+ trace(U(:,:,7,3)*J(:,:,7)*transpose(U(:,:,7,2))); 
    D(2,4)= trace(U(:,:,4,4)*J(:,:,4)*transpose(U(:,:,4,2)))+ trace(U(:,:,5,4)*J(:,:,5)*transpose(U(:,:,5,2)))+ trace(U(:,:,6,4)*J(:,:,6)*transpose(U(:,:,6,2)))+ trace(U(:,:,7,4)*J(:,:,7)*transpose(U(:,:,7,2))); 
    D(2,5)= trace(U(:,:,5,5)*J(:,:,5)*transpose(U(:,:,5,2)))+ trace(U(:,:,6,5)*J(:,:,6)*transpose(U(:,:,6,2)))+ trace(U(:,:,7,5)*J(:,:,7)*transpose(U(:,:,7,2)));
    D(2,6)= trace(U(:,:,6,6)*J(:,:,6)*transpose(U(:,:,6,2)))+ trace(U(:,:,7,6)*J(:,:,7)*transpose(U(:,:,7,2))); 
    D(2,7)= trace(U(:,:,7,7)*J(:,:,7)*transpose(U(:,:,7,2)));
  
    D(3,1)= trace(U(:,:,3,1)*J(:,:,3)*transpose(U(:,:,3,3)))+ trace(U(:,:,4,1)*J(:,:,4)*transpose(U(:,:,4,3)))+ trace(U(:,:,5,1)*J(:,:,5)*transpose(U(:,:,5,3)))+ trace(U(:,:,6,1)*J(:,:,6)*transpose(U(:,:,6,3)))+ trace(U(:,:,7,1)*J(:,:,7)*transpose(U(:,:,7,3)));
    D(3,2)= trace(U(:,:,3,2)*J(:,:,3)*transpose(U(:,:,3,3)))+ trace(U(:,:,4,2)*J(:,:,4)*transpose(U(:,:,4,3)))+ trace(U(:,:,5,2)*J(:,:,5)*transpose(U(:,:,5,3)))+ trace(U(:,:,6,2)*J(:,:,6)*transpose(U(:,:,6,3)))+ trace(U(:,:,7,2)*J(:,:,7)*transpose(U(:,:,7,3)));
    D(3,3)= trace(U(:,:,3,3)*J(:,:,3)*transpose(U(:,:,3,3)))+ trace(U(:,:,4,3)*J(:,:,4)*transpose(U(:,:,4,3)))+ trace(U(:,:,5,3)*J(:,:,5)*transpose(U(:,:,5,3)))+ trace(U(:,:,6,3)*J(:,:,6)*transpose(U(:,:,6,3)))+ trace(U(:,:,7,3)*J(:,:,7)*transpose(U(:,:,7,3)));
    D(3,4)= trace(U(:,:,4,4)*J(:,:,4)*transpose(U(:,:,4,3)))+ trace(U(:,:,5,4)*J(:,:,5)*transpose(U(:,:,5,3)))+ trace(U(:,:,6,4)*J(:,:,6)*transpose(U(:,:,6,3)))+ trace(U(:,:,7,4)*J(:,:,7)*transpose(U(:,:,7,3)));
    D(3,5)= trace(U(:,:,5,5)*J(:,:,5)*transpose(U(:,:,5,3)))+ trace(U(:,:,6,5)*J(:,:,6)*transpose(U(:,:,6,3)))+ trace(U(:,:,7,5)*J(:,:,7)*transpose(U(:,:,7,3)));
    D(3,6)= trace(U(:,:,6,6)*J(:,:,6)*transpose(U(:,:,6,3)))+ trace(U(:,:,7,6)*J(:,:,7)*transpose(U(:,:,7,3)));
    D(3,7)= trace(U(:,:,7,7)*J(:,:,7)*transpose(U(:,:,7,3)));
     
     
    D(4,1)= trace(U(:,:,4,1)*J(:,:,4)*transpose(U(:,:,4,4)))+ trace(U(:,:,5,1)*J(:,:,5)*transpose(U(:,:,5,4)))+ trace(U(:,:,6,1)*J(:,:,6)*transpose(U(:,:,6,4)))+ trace(U(:,:,7,1)*J(:,:,7)*transpose(U(:,:,7,4))); 
    D(4,2)= trace(U(:,:,4,2)*J(:,:,4)*transpose(U(:,:,4,4)))+ trace(U(:,:,5,2)*J(:,:,5)*transpose(U(:,:,5,4)))+ trace(U(:,:,6,2)*J(:,:,6)*transpose(U(:,:,6,4)))+ trace(U(:,:,7,2)*J(:,:,7)*transpose(U(:,:,7,4))); 
    D(4,3)= trace(U(:,:,4,3)*J(:,:,4)*transpose(U(:,:,4,4)))+ trace(U(:,:,5,3)*J(:,:,5)*transpose(U(:,:,5,4)))+ trace(U(:,:,6,3)*J(:,:,6)*transpose(U(:,:,6,4)))+ trace(U(:,:,7,3)*J(:,:,7)*transpose(U(:,:,7,4)));
    D(4,4)= trace(U(:,:,4,4)*J(:,:,4)*transpose(U(:,:,4,4)))+ trace(U(:,:,5,4)*J(:,:,5)*transpose(U(:,:,5,4)))+ trace(U(:,:,6,4)*J(:,:,6)*transpose(U(:,:,6,4)))+ trace(U(:,:,7,4)*J(:,:,7)*transpose(U(:,:,7,4)));
    D(4,5)= trace(U(:,:,5,5)*J(:,:,5)*transpose(U(:,:,5,4)))+ trace(U(:,:,6,5)*J(:,:,6)*transpose(U(:,:,6,4)))+ trace(U(:,:,7,5)*J(:,:,7)*transpose(U(:,:,7,4)));
    D(4,6)= trace(U(:,:,6,6)*J(:,:,6)*transpose(U(:,:,6,4)))+ trace(U(:,:,7,6)*J(:,:,7)*transpose(U(:,:,7,4))); 
    D(4,7)= trace(U(:,:,7,7)*J(:,:,7)*transpose(U(:,:,7,4)));
    
    D(5,1)= trace(U(:,:,5,1)*J(:,:,5)*transpose(U(:,:,5,5)))+ trace(U(:,:,6,1)*J(:,:,6)*transpose(U(:,:,6,5)))+ trace(U(:,:,7,1)*J(:,:,7)*transpose(U(:,:,7,5)));
    D(5,2)= trace(U(:,:,5,2)*J(:,:,5)*transpose(U(:,:,5,5)))+ trace(U(:,:,6,2)*J(:,:,6)*transpose(U(:,:,6,5)))+ trace(U(:,:,7,2)*J(:,:,7)*transpose(U(:,:,7,5)));
    D(5,3)= trace(U(:,:,5,3)*J(:,:,5)*transpose(U(:,:,5,5)))+ trace(U(:,:,6,3)*J(:,:,6)*transpose(U(:,:,6,5)))+ trace(U(:,:,7,3)*J(:,:,7)*transpose(U(:,:,7,5))); 
    D(5,4)= trace(U(:,:,5,4)*J(:,:,5)*transpose(U(:,:,5,5)))+ trace(U(:,:,6,4)*J(:,:,6)*transpose(U(:,:,6,5)))+ trace(U(:,:,7,4)*J(:,:,7)*transpose(U(:,:,7,5))); 
    D(5,5)= trace(U(:,:,5,5)*J(:,:,5)*transpose(U(:,:,5,5)))+ trace(U(:,:,6,5)*J(:,:,6)*transpose(U(:,:,6,5)))+ trace(U(:,:,7,5)*J(:,:,7)*transpose(U(:,:,7,5)));
    D(5,6)= trace(U(:,:,6,6)*J(:,:,6)*transpose(U(:,:,6,5)))+ trace(U(:,:,7,6)*J(:,:,7)*transpose(U(:,:,7,5))); 
    D(5,7)= trace(U(:,:,7,7)*J(:,:,7)*transpose(U(:,:,7,5)));
    
    D(6,1)= trace(U(:,:,6,1)*J(:,:,6)*transpose(U(:,:,6,6)))+ trace(U(:,:,7,1)*J(:,:,7)*transpose(U(:,:,7,6)));
    D(6,2)= trace(U(:,:,6,2)*J(:,:,6)*transpose(U(:,:,6,6)))+ trace(U(:,:,7,2)*J(:,:,7)*transpose(U(:,:,7,6)));
    D(6,3)= trace(U(:,:,6,3)*J(:,:,6)*transpose(U(:,:,6,6)))+ trace(U(:,:,7,3)*J(:,:,7)*transpose(U(:,:,7,6))); 
    D(6,4)= trace(U(:,:,6,4)*J(:,:,6)*transpose(U(:,:,6,6)))+ trace(U(:,:,7,4)*J(:,:,7)*transpose(U(:,:,7,6))); 
    D(6,5)= trace(U(:,:,6,5)*J(:,:,6)*transpose(U(:,:,6,6)))+ trace(U(:,:,7,5)*J(:,:,7)*transpose(U(:,:,7,6))); 
    D(6,6)= trace(U(:,:,6,6)*J(:,:,6)*transpose(U(:,:,6,6)))+ trace(U(:,:,7,6)*J(:,:,7)*transpose(U(:,:,7,6))); 
    D(6,7)= trace(U(:,:,7,7)*J(:,:,7)*transpose(U(:,:,7,6)));
    
    D(7,1)= trace(U(:,:,7,1)*J(:,:,7)*transpose(U(:,:,7,7)));
    D(7,2)= trace(U(:,:,7,2)*J(:,:,7)*transpose(U(:,:,7,7)));
    D(7,3)= trace(U(:,:,7,3)*J(:,:,7)*transpose(U(:,:,7,7)));
    D(7,4)= trace(U(:,:,7,4)*J(:,:,7)*transpose(U(:,:,7,7)));
    D(7,5)= trace(U(:,:,7,5)*J(:,:,7)*transpose(U(:,:,7,7)));
    D(7,6)= trace(U(:,:,7,6)*J(:,:,7)*transpose(U(:,:,7,7)));
    D(7,7)= trace(U(:,:,7,7)*J(:,:,7)*transpose(U(:,:,7,7)));
end 



function T = getTransformDH(a,d,alpha,q)
    ct = cos(q);
    st = sin(q);
    cb = cos(alpha);
    sb = sin(alpha);
    
    T = [ ct, -st*cb,  st*sb, a*ct;
          st,  ct*cb, -ct*sb, a*st;
          0, sb, cb, d;
          0, 0, 0, 1 ];
end
